simulink model "RedCrane_Merged_control_05032025"  (R2024b)
settings: Solver=VariableStepAuto  StartTime=0.0  StopTime=20  RelTol=1e-4
model workspace (MATLAB code in the model file):
  | %% Geometric properties
  | 
  | %Basic geometry width
  | w0 = 0.07;
  | w1 = w0/4;
  | l_RJ = 0.277; %2.1*w0;
  | r_RJ = 0.030;
  | 
  | %Column geometry
  | L_Column = 1.5655; %2;
  | eta_B = -0.25;
  | zeta_B = L_Column;
  | eta_D = -0.365; %0.25;
  | zeta_D = 1.4805; %1.5;
  | eta_J = 0.200; % 0.25;
  | zeta_J = 0.1195; %0.25;
  | 
  | %Column - Main boom link
  | l_DE = 0.490; % 0.5;
  | l_FE = 0.170; % 0.4;
  | 
  | %Main boom geometry
  | L_Mboom = 2.400; % 2;
  | eta_C = 2.400; % 2;
  | zeta_C = 0.070; % 0.25;
  | eta_F = 0.340; % 0.6;
  | zeta_F = 0.010; % -0.25;
  | eta_G = 2.365; % 1.75;
  | zeta_G = 0.235; % -0.25;
  | eta_K = 0.750; % 1;
  | zeta_K = 0.045; % -0.25;
  | 
  | %Main boom-Jib boom link
  | l_GH = 0.490; % 0.5;
  | l_IH = 0.220; % 0.4;
  | 
  | %Jib boom geometry
  | L_Jib_boom = 2.429; % 2;
  | eta_I = 0.280; % 0.5;
  | zeta_I = 0.005; % -0.25;
  | eta_TP = L_Jib_boom;
  | zeta_TP = 0;
  | 
  | % Winch
  | r_W = 0.205/2;
  | L_W = 0.191;
  | eta_W = 0.28722;
  | zeta_W = -0.29926;
  | beta_W = -0.335;
  | 
  | % Mounting plate
  | eta_MP = -0.0249;
  | zeta_MP = -0.17479;
  | beta_MP = 0;
  | 
  | % Pulley
  | r_P = 0.210/2; % Radius pulley
  | eta_P = 2.140;
  | zeta_P = -0.0506;
  | beta_P = -0.0;
  | 
  | %Roller
  | r_RO = 0.055/2; % Radius roller over
  | r_RU = 0.046/2; % Radius roller under
  | eta_RO = 0.306;
  | zeta_RO = 0.12510;
  | 
  | %Mounting
  | L_M = 1; %m
  | W_M = 1; %m
  | H_M = 1; %m
  | eta_M = 0; %m
  | zeta_M = -0.5; %m
  | beta_M = 0; %m
  | 
  | %Ground
  | L_ground = 6; %m
  | W_ground = 4; %m
  | H_ground = 0.01; %m
  | eta_ground = 1.5; %m
  | zeta_ground = -0.5; %m
  | beta_ground = 0; %m
  | 
  | 
  | %% Mass properties (Mass and center of mass)
  | column_mass = 239.4; % kg
  | column_COM = [-0.1007, 0.0001, 0.4351]; % m
  | 
  | MainBoom_mass = 216.5; % kg
  | MainBoom_COM = [1.134, 0.1674, -0.0018]; % m
  | 
  | JibBoom_mass = 842.2; % kg
  | JibBoom_COM = [0.9806, 0.1814, -0.2939]; % m
  | 
  | % Dogbone
  | E2F_mass = 7.076*2; % kg
  | E2F_COM = [0.0817, 0, 0]; % m
  | 
  | D2E_mass = 6.426*2; % kg
  | D2E_COM = [0.245, 0, 0]; % m
  | 
  | G2H_mass = 6.426*2; % kg
  | G2H_COM = [0.245, 0, 0]; % m
  | 
  | H2I_mass = 22.05; % kg
  | H2I_COM = [0.1206, 0, 0]; % m
  | 
  | % Main cylinder
  | MainC_bottom_mass = 57.9561; % kg
  | MainC_bottom_COM = [0.0081, -0.001, 0.4125]; % m
  | 
  | MainC_rod_mass = 43.93; % kg
  | MainC_rod_COM = [0, 0, -0.4290]; % m
  | 
  | % Jib cylinder
  | JibC_bottom_mass = 55.7738; % kg
  | JibC_bottom_COM = [0.0038, 0.0022, 0.4468]; % m
  | 
  | JibC_rod_mass = 45.8854; % kg
  | JibC_rod_COM = [0, 0, -0.4694]; % m
  | 
  | % Winch
  | Winch_mass = 54; % kg
  | Winch_COM = [0, 0, 0]; % m
  | 
  | 
  | %% Inertia properties (Moments of inertia and products of inertia)
  | 
  | column_MOI = [109, 114, 9.009]; % kg*m^2
  | column_POI = [0.0319, -21.59, -0.0113]; % kg*m^2
  | 
  | MainBoom_MOI = [6.5, 160.3, 160]; % kg*m^2
  | MainBoom_POI = [0.0666, 0.1093, 8.016]; % kg*m^2
  | 
  | JibBoom_MOI = [31.75, 566.3, 573.1]; % kg*m^2
  | JibBoom_POI = [-0.0237, -11.42, 9.588]; % kg*m^2
  | 
  | % Dogbone
  | E2F_MOI = [0.0111, 0.0546, 0.0587]; % kg*m^2
  | E2F_POI = [0, -0.0089, 0]; % kg*m^2
  | 
  | D2E_MOI = [0.0069, 0.2419, 0.2485]; % kg*m^2
  | D2E_POI = [0, 0, 0]; % kg*m^2
  | 
  | G2H_MOI = [0.0069, 0.2419, 0.2485]; % kg*m^2
  | G2H_POI = [0, 0, 0]; % kg*m^2
  | 
  | H2I_MOI = [0.2636, 0.4184, 0.1901]; % kg*m^2
  | H2I_POI = [0, 0, 0]; % kg*m^2
  | 
  | 
  | % Main cylinder
  | MainC_bottom_MOI = [7.2059, 7.2304, 0.3979]; % kg*m^2
  | MainC_bottom_POI = [-0.0126, -0.1802, 0.0002]; % kg*m^2
  | 
  | MainC_rod_MOI = [6.0014, 5.9633, 0.1401]; % kg*m^2
  | MainC_rod_POI = [0, -0.0001, 0]; % kg*m^2
  | 
  | % Jib cylinder
  | JibC_bottom_MOI = [8.3780, 8.3476, 0.3607]; % kg*m^2
  | JibC_bottom_POI = [-0.0119, -0.1037, 0.0033]; % kg*m^2
  | 
  | JibC_rod_MOI = [7.4245, 7.3864, 0.1401]; % kg*m^2
  | JibC_rod_POI = [0, -0.0001, 0]; % kg*m^2
  | 
  | % Winch
  | I_W_xx = (1/4)*Winch_mass*r_W^2 + (1/12)*Winch_mass*L_W^2;
  | I_W_yy = (1/4)*Winch_mass*r_W^2 + (1/12)*Winch_mass*L_W^2;
  | I_W_zz = (1/2)*Winch_mass*r_W^2;
  | 
  | Winch_MOI = [I_W_xx, I_W_yy, I_W_zz]; % kg*m^2
  | Winch_POI = [0, 0, 0]; % kg*m^2
  | 
  | 
  | %% Hydraulics
  | 
  | %-------------Cylinder---------------------
  | 
  | % Main cylinder
  | D_piston_MainC = 160; %mm dimater of piston side
  | L_piston_MainC = 65; %66.2;%mm length from joint to buttom of piston side
  | D_rod_MainC = 100; %mm diamter of cylinder rod
  | L_rod_MainC = 978; %990;%mm length from bottom of rod to joint
  | A_piston_MainC = pi/4*D_piston_MainC^2; % mm^2 area of piston side
  | A_rod_MainC = pi/4*D_rod_MainC^2; % mm^2 area of rod
  | A_rodside_MainC = A_piston_MainC-A_rod_MainC; % mm^2 area of rod side
  | L_barrel_MainC = 945-L_piston_MainC; %mm
  | stroke_MainC = 0.75; %m
  | initial_pos_Main = 0.3; %m
  | initial_Pa_Main = 17;%Bar
  | 
  | % Jib cylinder
  | D_piston_JibC = 150; %mm dimater of piston side
  | L_piston_JibC = 65; %66.2;%mm length from joint to buttom of piston side
  | D_rod_JibC = 100; %mm diamter of cylinder rod
  | L_rod_JibC = 1089.5; %1105.5;%mm length from bottom of rod to joint
  | A_piston_JibC = pi/4*D_piston_JibC^2; % mm^2 area of piston side
  | A_rod_JibC = pi/4*D_rod_JibC^2; % mm^2 area of rod
  | A_rodside_JibC = A_piston_JibC-A_rod_JibC; % mm^2 area of rod side
  | L_barrel_JibC = 1050-L_piston_JibC; %mm
  | stroke_JibC = 0.85; %m
  | initial_pos_Jib = 0.4; %m
  | initial_Pa_Jib = 1;%Bar
  | initial_Pb_Jib = 67;%Bar
  | 
  | % winch
  | poly_b = [1.762740809095876e+02,-44.442169999547330];
  | poly_c = [1.901177983521692e+02,-1.484122102902541e+02];
  | angle_b = poly_b(1)*initial_pos_Main + poly_b(2);
  | angle_c = poly_c(1)*initial_pos_Jib + poly_c(2);
  | angle_w = -90 - angle_c - angle_b;
  | 
  | %Motor
  | DM = 200; %Displacement cm^3/rev
  | GR = 5.04; % Gear ratio 1:5,04
  | 
  | 
  | % ------------------CBV-------------------
  | 
  | % Main
  | pCr_Main = 25;%Bar
  | dp_open_Main = 300;%Bar
  | 
  | % Jib
  | alpha = 4.25;
  | pCr_Jib_A = 211;%Bar
  | dp_open_Jib_A = 300;%Bar
  | pCr_Jib_B = 211;%Bar
  | dp_open_Jib_B = 300;%Bar
  | 
  | %-------------------DCV-----------------------
  | Cd = 0.64;
  | Q_rat = 30/6e4;
  | dp_2 = 6e5;
  | dp_1 = 1e5;
  | roh = 850;
  | 
  | % Main dcv
  | dead_up_Main = 0.071;
  | dead_down_Main = 0.126;
  | 
  | % Jib dcv
  | dead_up_Jib = 0.037;
  | dead_down_Jib = 0.126;
  | 
  | Ad2 = Q_rat/(Cd*sqrt(2/roh*dp_2))*1e6; %mm
  | Ad1_1 = Q_rat/(Cd*sqrt(2/roh*dp_1))*1e6;
  | Ad1_0 = Q_rat/(Cd*sqrt(2/roh*dp_1))*1e6*0;
  | 
  | Ad1_Main_up = Q_rat/(Cd*sqrt(2/roh*dp_1))*1e6*dead_up_Main;
  | Ad1_Main_down = Q_rat/(Cd*sqrt(2/roh*dp_1))*1e6*dead_down_Main;
  | Ad1_Jib_up = Q_rat/(Cd*sqrt(2/roh*dp_1))*1e6*dead_up_Jib;
  | Ad1_Jib_down = Q_rat/(Cd*sqrt(2/roh*dp_1))*1e6*dead_down_Jib;
undefined symbols (not defined in the file or in its folder): dead_down_m, dead_up_m, X, Y, Z
libraries: sm_lib x171, fl_lib x65, nesl_utility x48, SimscapeFluids_lib x27, sdl_lib x1
(part 8 of 8)

== matlab function RedCrane_Merged_control_05032025/Jib Control/MATLAB Function ==
  data: t input; x output; x_dot output; initial_pos_Jib parameter
function [x, x_dot] = fcn(t,initial_pos_Jib)

amplitude = 0.1;
median = initial_pos_Jib+amplitude;
frekvens = 0.05; %1/20
 
x = median - amplitude * cos(2*pi*frekvens*t);
x_dot = amplitude*2*pi*frekvens*sin(2*pi*frekvens*t);

== matlab function RedCrane_Merged_control_05032025/Jib Control/MATLAB Function1 ==
  data: x_dot input; U_FF output; Pa input; Pb input; Ps input; A_piston_JibC parameter; A_rodside_JibC parameter; Q_adj output; Q_ref output; dead_up_Jib parameter; dead_down_Jib parameter
function [U_FF,Q_adj,Q_ref] = fcn(x_dot, Pa, Pb, Ps, A_piston_JibC,A_rodside_JibC,dead_up_Jib,dead_down_Jib)

dp_0 = 6e5; %Pa
Q_0 = 30/60000; %m^3/s

if x_dot >= 0
    dp = (Ps-Pa)*1e5;
    if dp <=100
        dp = 100;
    end
    Q_ref = A_piston_JibC*1e-6 * x_dot;
    Q_adj = Q_ref * sqrt(dp_0/dp);
    U_FF = Q_adj/Q_0;
    U_FF = U_FF*(1-dead_up_Jib);
elseif x_dot < 0
    dp = (Ps-Pb)*1e5;
    if dp <=100
        dp = 100;
    end
    Q_ref = A_rodside_JibC*1e-6 * x_dot;
    Q_adj = Q_ref * sqrt(dp_0/dp);
    U_FF = Q_adj/Q_0;
    U_FF = U_FF*(1-dead_down_Jib);
else
    U_FF = 0;
    Q_ref = 0;
    Q_adj = 0;
end

Q_ref = Q_ref*60000;
Q_adj = Q_adj*60000;

== matlab function RedCrane_Merged_control_05032025/Jib Control/MATLAB Function2 ==
  data: U_PID input; U_FF input; U output; dead_down_Jib parameter; dead_up_Jib parameter
function U = fcn(U_PID,U_FF, dead_down_Jib, dead_up_Jib)
U_adj = U_FF+U_PID;
if U_PID >= 0
    U = U_adj+dead_up_Jib;
elseif U_PID < 0
    U = U_adj-dead_down_Jib;
else
    U=0;
end

== matlab function RedCrane_Merged_control_05032025/Jib cylinder/Subsystem3/CBV_opening_B ==
  data: pB input; uCBV output; pBm input; pA input; pCr_Jib_B parameter; dp_open_Jib_B parameter; alpha parameter
function uCBV = fcn(pB,pBm,pA,pCr_Jib_B, dp_open_Jib_B, alpha)

uCBV = (alpha*pA + pBm - pCr_Jib_B - (alpha + 1)*pB)/dp_open_Jib_B;
%uCBV = (alpha*pB + pAm - pCr)/dpopen; %vented
%uCBV = 0.25;
if uCBV < 0
    uCBV = 0;
elseif uCBV > 1
    uCBV = 1;
end

== matlab function RedCrane_Merged_control_05032025/Jib cylinder/Subsystem3/CBV_opening_A ==
  data: pB input; uCBV output; pAm input; pA input; pCr_Jib_A parameter; dp_open_Jib_A parameter; alpha parameter
function uCBV = fcn(pB,pAm,pA,pCr_Jib_A, dp_open_Jib_A, alpha)

uCBV = (alpha*pB + pAm - pCr_Jib_A - (alpha + 1)*pA)/dp_open_Jib_A;
%uCBV = (alpha*pB + pAm - pCr)/dpopen; %vented
%uCBV = 0.25;
if uCBV < 0
    uCBV = 0;
elseif uCBV > 1
    uCBV = 1;
end

== matlab function RedCrane_Merged_control_05032025/Main cylinder/Subsystem3/CBV_opening_A ==
  data: pB input; uCBV output; pA input; pCr_Main parameter; dp_open_Main parameter
function uCBV = fcn(pB,pA,pCr_Main, dp_open_Main)
% uCBV = (alpha*pB + pAm - pCr - (alpha + 1)*pA)/dpopen;
uCBV = (pB - pCr_Main- pA)/dp_open_Main; %vented
%uCBV = 0.25;
if uCBV < 0
    uCBV = 0;
elseif uCBV > 1
    uCBV = 1;
end

== matlab function RedCrane_Merged_control_05032025/Main Control/MATLAB Function ==
  data: t input; x output; x_dot output; initial_pos_Main parameter
function [x, x_dot] = fcn(t,initial_pos_Main)

amplitude = 0.1;
median = initial_pos_Main+amplitude;
frekvens = 0.05; % 1/20

x = median - amplitude * cos(2*pi*frekvens*t);
x_dot = amplitude*2*pi*frekvens*sin(2*pi*frekvens*t);

== matlab function RedCrane_Merged_control_05032025/Main cylinder/Subsystem2/uAT ==
  data: U input; u output; dead_up_Main parameter; dead_down_Main parameter
function u = fcn(U,dead_up_Main, dead_down_Main)
if U < -dead_up_Main
    u=0;
elseif U <= 0
    u = dead_down_Main-abs(U);
elseif U <= dead_down_Main
    u = dead_down_Main;
elseif U >dead_down_Main
    u= (U-dead_down_Main)/(1-dead_down_Main)+dead_down_Main;
else
    u = 0;
end

== matlab function RedCrane_Merged_control_05032025/Main cylinder/Subsystem2/uBT ==
  data: U input; u output; dead_up_Main parameter; dead_down_Main parameter
function u = fcn(U,dead_up_Main, dead_down_Main)
if U < -dead_down_Main
    u=0;
elseif U <= 0
    u = dead_up_Main-abs(U);
elseif U <= dead_up_Main
    u = dead_up_Main;
elseif U >dead_up_Main
    u= (U-dead_up_Main)/(1-dead_up_Main)+dead_up_Main;
else
    u = 0;
end

== matlab function RedCrane_Merged_control_05032025/Main Control/MATLAB Function1 ==
  data: x_dot input; U_FF output; Pa input; Pb input; Ps input; A_piston_MainC parameter; A_rodside_MainC parameter; Q_adj output; Q_ref output; dead_up_Main parameter; dead_down_Main parameter
function [U_FF,Q_adj,Q_ref] = fcn(x_dot, Pa, Pb, Ps, A_piston_MainC, A_rodside_MainC, dead_up_Main, dead_down_Main)

dp_0 = 6e5; %Pa
Q_0 = 30/60000; %m^3/s

if x_dot >= 0
    dp = (Ps-Pa)*1e5;
    if dp <=100
        dp = 100;
    end
    Q_ref = A_piston_MainC*1e-6 * x_dot;
    Q_adj = Q_ref * sqrt(dp_0/dp);
    U_FF = Q_adj/Q_0;
    U_FF = U_FF*(1-dead_up_Main);
elseif x_dot < 0
    dp = (Ps-Pb)*1e5;
    if dp <=100
        dp = 100;
    end
    Q_ref = A_rodside_MainC*1e-6 * x_dot;
    Q_adj = Q_ref * sqrt(dp_0/dp);
    U_FF = Q_adj/Q_0;
    U_FF = U_FF*(1-dead_down_Main);
else
    U_FF = 0;
    Q_ref = 0;
    Q_adj = 0;
end

Q_ref = Q_ref*60000;
Q_adj = Q_adj*60000;

== matlab function RedCrane_Merged_control_05032025/Main Control/MATLAB Function2 ==
  data: U_PID input; U_FF input; U output; dead_down_Main parameter; dead_up_Main parameter
function U = fcn(U_PID,U_FF, dead_down_Main, dead_up_Main)
U_adj = U_FF+U_PID;
if U_PID >= 0
    U = U_adj+dead_up_Main;
elseif U_PID < 0
    U = U_adj-dead_down_Main;
else
    U=0;
end
